simulink model "NumSim_standard_eVTOL"  (R2024b)
settings: Solver=ode14x  StartTime=0.0  StopTime=250  FixedStep=0.005  RelTol=1e-3
values from neighbouring files (symbols this model uses):
  aDl =     [initdata.mat]
  aDr =     [initdata.mat]
  aDyn =     [initdata.mat]
  Airport = init_airport('PHNL')    [initdata_HIL_eVTOL.m]
  aLat =     [initdata.mat]
  aLon =     [initdata.mat]
  D = Prop.D    [EOM_dt_MC.m]    (also in EOM_get_alf_dt_de_prop_evtol.m = CD * QS)
  dt0 = X(2)    [EOM_get_alf_dt_de_prop_evtol.m]    (also in initdata.mat = 0.258252593971; initdata_HIL_eVTOL.m = EOM_dt_MC)
  EAS0 = TAS0 / EAS2TAS    [initdata_HIL_eVTOL.m]
  FCS = init_FCS    [initdata_HIL_eVTOL.m]
  General = init_layoutdata    [EOM_dt_MC.m]    (also in build_optimized_CA.m; initdata.mat = ; initdata_HIL_eVTOL.m)
  h0 = Con(1)    [EOM_get_alf_dt_de_prop_evtol.m]    (also in initdata.mat = 450; initdata_HIL_eVTOL.m = 50)
  mass = Con(3)    [EOM_get_alf_dt_de_prop_evtol.m]    (also in initdata.mat = 2255.54; initdata_HIL_eVTOL.m = 7)
  Motor = init_motor_evtol    [EOM_dt_MC.m]    (also in initdata.mat = []; initdata_HIL_eVTOL.m)
  Prop = init_propeller_evtol_new    [EOM_dt_MC.m]    (also in initdata_HIL_eVTOL.m)
  R2D = 180/pi    (= 57.2957795131)    [EOM_get_alf_dt_de_prop_evtol.m]    (also in init_FCS.m; init_aerodata_evtol.m; init_airport.m; initdata.mat)
  theta0 = -0.0510981441662    [initdata.mat]
undefined symbols (not defined in the file or in its folder): A1, aDa, aDe, asbhl20env, B1, C1, de0, Earth, Environment, InitData, Kd, Kp, magnitude, Tc, WGS84
libraries: simulink_extras x26, simulink x18, slpidlib x14, vrlib x8, matrix_library x6, sharedutil x6, sharedtransform x5, aerolibwindfilters x4, aerolibatmos2 x3, aerolibobsolete x2, aerolibactuator x2, aerolibasang x2
(part 3 of 7)

== system NumSim_standard_eVTOL/Energy & Power/thrust_5/Motor ==
  P_shaft : Inport
  dt : Inport  Port=2
  V : Inport  Port=3
  rpm0 : Inport  Port=4
  rho : Inport  Port=5
  rpm_grid : Inport  Port=6
  Constant : Constant  Value=Motor.Ue
  Constant1 : Constant  Value=Motor.Re
  Constant2 : Constant  Value=Motor.Rm
  Constant3 : Constant  Value=Motor.KE
  Constant4 : Constant  Value=Motor.KT  VectorParams1D=off
  Constant5 : Constant  Value=Motor.Im0
  Constant6 : Constant  Value=0
  D^5 : Constant  Value=5
  Diameter : Constant  Value=Prop.D
  Diameter1 : Constant  Value=Prop.D
  Divide : Product  Inputs=*//
  Ea : Sum  Inputs=+-
  Gain1 : Gain  Gain=30/pi
  Gain2 : Gain  Gain=pi/30
  Gain3 : Gain  Gain=1/60
  Gain4 : Gain  Gain=1/(2*pi)
  Im : Sum
  Integrator : Integrator  InitialConditionSource=external  InitialCondition=600
  Ix : Constant  Value=Prop.Ix
  J : Product  Inputs=*//
  Manual Switch : ManualSwitch
  Math Function : Math  Operator=magnitude^2  SignedPower=on
  Math Function3 : Math  Operator=pow  SignedPower=on
  Math Function4 : Math  Operator=pow  SignedPower=on
  Memory : Memory  InitialCondition=0.1
  N(rpm) : Product  Inputs=*/
  N(rpm)1 : Product  Inputs=/*
  P Scope : Scope  NumInputPorts=2
  P_sp : Product  Inputs=4
  Product1 : Product
  Product2 : Product
  Q : Product  Inputs=4
  RPM 5 : Scope
  Saturation : Saturate  UpperLimit=1047.2  LowerLimit=0.1
  Scope : Scope
  Sum : Sum  Inputs=|+-
  Ueo : Product
  Um : Sum  Inputs=+-
  get CP : Lookup_n-D  BreakpointsForDimension1=Prop.J  BreakpointsForDimension2=Prop.rpm_grid  IndexSearchMethod=Linear search  BeginIndexSearchUsingPreviousIndexResult=on  Table=Prop.CP  RndMeth=Simplest
      settings: InputPortMap=u0,u1
  "n^3 " : Constant  Value=3
  rpm : Outport  VectorParamsAs1DForOutWhenUnconnected=off
  wires:
  Saturation/1 -> Gain1/1, Divide/2
  Gain2/1 -> Integrator/2
  rpm0/1 -> Manual Switch/1
  Gain1/1 -> rpm/1, RPM 5/1  "rpm"
  Sum/1 -> Divide/1  "DP"
  Divide/1 -> Integrator/1  "omega_dot"
  dt/1 -> Ueo/1
  Integrator/1 -> Saturation/1  "omega"
  P_sp/1 -> Scope/1, P Scope/1, Sum/1
  P_shaft/1 -> P Scope/2, Sum/2
  Ix/1 -> Divide/3
  Constant/1 -> Ueo/2
  Ueo/1 -> Um/1
  Product1/1 -> Um/2
  Constant1/1 -> Product1/1
  Um/1 -> Ea/1
  Product2/1 -> Ea/2
  Constant2/1 -> Product2/1
  Ea/1 -> N(rpm)/1
  Constant3/1 -> N(rpm)/2
  Diameter/1 -> J/2
  V/1 -> J/1
  N(rpm)/1 -> Gain3/1
  J/1 -> get CP/1
  rpm_grid/1 -> get CP/2
  Gain4/1 -> Q/2  "CQ"
  D^5/1 -> Math Function4/2
  Diameter1/1 -> Math Function4/1
  Math Function/1 -> Q/3  "n^2"
  Q/1 -> N(rpm)1/2
  Constant4/1 -> N(rpm)1/1
  N(rpm)1/1 -> Im/1
  Constant5/1 -> Im/2
  Im/1 -> Product1/2, Product2/2
  rho/1 -> Q/1, P_sp/3  "rho"
  Math Function3/1 -> P_sp/2  "n^3"
  "n^3 "/1 -> Math Function3/2
  Math Function4/1 -> Q/4, P_sp/4  "D^5"
  get CP/1 -> Gain4/1, P_sp/1  "CP"
  Constant6/1 -> Manual Switch/2
  Manual Switch/1 -> Gain2/1
  Gain3/1 -> Memory/1  "rps"
  Memory/1 -> J/3, Math Function3/1, Math Function/1

== system NumSim_standard_eVTOL/Energy & Power/thrust_5/Propeller  ==
  rpm : Inport
  V : Inport  Port=2
  rho : Inport  Port=3
  D^5 : Constant  Value=5
  Diameter : Constant  Value=Prop.D
  Divide : Product  Inputs=4
  Divide2 : Product  Inputs=4
  Divide3 : Product  Inputs=**/
  Gain : Gain  Gain=1/60
  Math Function : Math  Operator=magnitude^2  SignedPower=on
  Math Function1 : Math  Operator=magnitude^2  SignedPower=on
  Math Function2 : Math  Operator=magnitude^2  SignedPower=on
  Math Function3 : Math  Operator=pow  SignedPower=on
  Math Function4 : Math  Operator=pow  SignedPower=on
  Scope{,1..4} (5 alike) : Scope
  Subsystem : Subsystem
  get CP : Lookup_n-D  BreakpointsForDimension1=Prop.J  BreakpointsForDimension2=Prop.rpm_grid  IndexSearchMethod=Linear search  BeginIndexSearchUsingPreviousIndexResult=on  Table=Prop.CP  RndMeth=Simplest
      settings: InputPortMap=u0,u1
  get CT : Lookup_n-D  BreakpointsForDimension1=Prop.J  BreakpointsForDimension2=Prop.rpm_grid  IndexSearchMethod=Linear search  BeginIndexSearchUsingPreviousIndexResult=on  Table=Prop.CT  RndMeth=Simplest
      settings: InputPortMap=u0,u1
  "n^3 " : Constant  Value=3
  P_plr (w) : Outport  VectorParamsAs1DForOutWhenUnconnected=off
  T (N) : Outport  Port=2  VectorParamsAs1DForOutWhenUnconnected=off
  eta_p : Outport  Port=3  VectorParamsAs1DForOutWhenUnconnected=off
  wires:
  Divide2/1 -> P_plr (w)/1, Scope/1
  Divide3/1 -> eta_p/1  "eta_p"
  D^5/1 -> Math Function4/2
  Math Function4/1 -> Divide2/4
  "n^3 "/1 -> Math Function3/2
  Math Function3/1 -> Divide2/3
  get CP/1 -> Divide3/3, Divide2/1, Scope3/1
  Subsystem/1(J) -> Scope2/1, get CT/1, Divide3/1, get CP/1
  Divide/1 -> Scope1/1, T (N)/1
  Math Function2/1 -> Divide/4  "D^4"
  Math Function1/1 -> Math Function2/1
  Diameter/1 -> Math Function1/1, Math Function4/1
  Math Function/1 -> Divide/3  "n^2"
  Gain/1 -> Math Function3/1, Math Function/1
  rho/1 -> Divide/2, Divide2/2
  get CT/1 -> Divide3/2, Divide/1, Scope4/1
  V/1 -> Subsystem/1(V)
  rpm/1 -> get CP/2, get CT/2, Gain/1, Subsystem/2(rpm)

== system NumSim_standard_eVTOL/Energy & Power/thrust_6/Motor ==
  P_shaft : Inport
  dt : Inport  Port=2
  V : Inport  Port=3
  rpm0 : Inport  Port=4
  rho : Inport  Port=5
  rpm_grid : Inport  Port=6
  Constant : Constant  Value=Motor.Ue
  Constant1 : Constant  Value=Motor.Re
  Constant2 : Constant  Value=Motor.Rm
  Constant3 : Constant  Value=Motor.KE
  Constant4 : Constant  Value=Motor.KT  VectorParams1D=off
  Constant5 : Constant  Value=Motor.Im0
  Constant6 : Constant  Value=0
  D^5 : Constant  Value=5
  Diameter : Constant  Value=Prop.D
  Diameter1 : Constant  Value=Prop.D
  Divide : Product  Inputs=*//
  Ea : Sum  Inputs=+-
  Gain1 : Gain  Gain=30/pi
  Gain2 : Gain  Gain=pi/30
  Gain3 : Gain  Gain=1/60
  Gain4 : Gain  Gain=1/(2*pi)
  Im : Sum
  Integrator : Integrator  InitialConditionSource=external  InitialCondition=600
  Ix : Constant  Value=Prop.Ix
  J : Product  Inputs=*//
  Manual Switch : ManualSwitch
  Math Function : Math  Operator=magnitude^2  SignedPower=on
  Math Function3 : Math  Operator=pow  SignedPower=on
  Math Function4 : Math  Operator=pow  SignedPower=on
  Memory : Memory  InitialCondition=0.1
  N(rpm) : Product  Inputs=*/
  N(rpm)1 : Product  Inputs=/*
  P Scope : Scope  NumInputPorts=2
  P_sp : Product  Inputs=4
  Product1 : Product
  Product2 : Product
  Q : Product  Inputs=4
  RPM 6 : Scope
  Saturation : Saturate  UpperLimit=1047.2  LowerLimit=0.1
  Scope : Scope
  Sum : Sum  Inputs=|+-
  Ueo : Product
  Um : Sum  Inputs=+-
  get CP : Lookup_n-D  BreakpointsForDimension1=Prop.J  BreakpointsForDimension2=Prop.rpm_grid  IndexSearchMethod=Linear search  BeginIndexSearchUsingPreviousIndexResult=on  Table=Prop.CP  RndMeth=Simplest
      settings: InputPortMap=u0,u1
  "n^3 " : Constant  Value=3
  rpm : Outport  VectorParamsAs1DForOutWhenUnconnected=off
  wires:
  Saturation/1 -> Gain1/1, Divide/2
  Gain2/1 -> Integrator/2
  rpm0/1 -> Manual Switch/1
  Gain1/1 -> rpm/1, RPM 6/1  "rpm"
  Sum/1 -> Divide/1  "DP"
  Divide/1 -> Integrator/1  "omega_dot"
  dt/1 -> Ueo/1
  Integrator/1 -> Saturation/1  "omega"
  P_sp/1 -> Scope/1, P Scope/1, Sum/1
  P_shaft/1 -> P Scope/2, Sum/2
  Ix/1 -> Divide/3
  Constant/1 -> Ueo/2
  Ueo/1 -> Um/1
  Product1/1 -> Um/2
  Constant1/1 -> Product1/1
  Um/1 -> Ea/1
  Product2/1 -> Ea/2
  Constant2/1 -> Product2/1
  Ea/1 -> N(rpm)/1
  Constant3/1 -> N(rpm)/2
  Diameter/1 -> J/2
  V/1 -> J/1
  N(rpm)/1 -> Gain3/1
  J/1 -> get CP/1
  rpm_grid/1 -> get CP/2
  Gain4/1 -> Q/2  "CQ"
  D^5/1 -> Math Function4/2
  Diameter1/1 -> Math Function4/1
  Math Function/1 -> Q/3  "n^2"
  Q/1 -> N(rpm)1/2
  Constant4/1 -> N(rpm)1/1
  N(rpm)1/1 -> Im/1
  Constant5/1 -> Im/2
  Im/1 -> Product1/2, Product2/2
  rho/1 -> Q/1, P_sp/3  "rho"
  Math Function3/1 -> P_sp/2  "n^3"
  "n^3 "/1 -> Math Function3/2
  Math Function4/1 -> Q/4, P_sp/4  "D^5"
  get CP/1 -> Gain4/1, P_sp/1  "CP"
  Constant6/1 -> Manual Switch/2
  Manual Switch/1 -> Gain2/1
  Gain3/1 -> Memory/1  "rps"
  Memory/1 -> J/3, Math Function3/1, Math Function/1

== system NumSim_standard_eVTOL/Energy & Power/thrust_6/Propeller  ==
  rpm : Inport
  V : Inport  Port=2
  rho : Inport  Port=3
  D^5 : Constant  Value=5
  Diameter : Constant  Value=Prop.D
  Divide : Product  Inputs=4
  Divide2 : Product  Inputs=4
  Divide3 : Product  Inputs=**/
  Gain : Gain  Gain=1/60
  Math Function : Math  Operator=magnitude^2  SignedPower=on
  Math Function1 : Math  Operator=magnitude^2  SignedPower=on
  Math Function2 : Math  Operator=magnitude^2  SignedPower=on
  Math Function3 : Math  Operator=pow  SignedPower=on
  Math Function4 : Math  Operator=pow  SignedPower=on
  Scope{,1..4} (5 alike) : Scope
  Subsystem : Subsystem
  get CP : Lookup_n-D  BreakpointsForDimension1=Prop.J  BreakpointsForDimension2=Prop.rpm_grid  IndexSearchMethod=Linear search  BeginIndexSearchUsingPreviousIndexResult=on  Table=Prop.CP  RndMeth=Simplest
      settings: InputPortMap=u0,u1
  get CT : Lookup_n-D  BreakpointsForDimension1=Prop.J  BreakpointsForDimension2=Prop.rpm_grid  IndexSearchMethod=Linear search  BeginIndexSearchUsingPreviousIndexResult=on  Table=Prop.CT  RndMeth=Simplest
      settings: InputPortMap=u0,u1
  "n^3 " : Constant  Value=3
  P_plr (w) : Outport  VectorParamsAs1DForOutWhenUnconnected=off
  T (N) : Outport  Port=2  VectorParamsAs1DForOutWhenUnconnected=off
  eta_p : Outport  Port=3  VectorParamsAs1DForOutWhenUnconnected=off
  wires:
  Divide2/1 -> P_plr (w)/1, Scope/1
  Divide3/1 -> eta_p/1  "eta_p"
  D^5/1 -> Math Function4/2
  Math Function4/1 -> Divide2/4
  "n^3 "/1 -> Math Function3/2
  Math Function3/1 -> Divide2/3
  get CP/1 -> Divide3/3, Divide2/1, Scope3/1
  Subsystem/1(J) -> Scope2/1, get CT/1, Divide3/1, get CP/1
  Divide/1 -> Scope1/1, T (N)/1
  Math Function2/1 -> Divide/4  "D^4"
  Math Function1/1 -> Math Function2/1
  Diameter/1 -> Math Function1/1, Math Function4/1
  Math Function/1 -> Divide/3  "n^2"
  Gain/1 -> Math Function3/1, Math Function/1
  rho/1 -> Divide/2, Divide2/2
  get CT/1 -> Divide3/2, Divide/1, Scope4/1
  V/1 -> Subsystem/1(V)
  rpm/1 -> get CP/2, get CT/2, Gain/1, Subsystem/2(rpm)

== system NumSim_standard_eVTOL/Environment/Wind Models/Dryden Wind Turbulence Model (Continuous (+q -r)) ==
  Altitude : Inport  Unit=m
  Airspeed : Inport  Port=2  Unit=m/s
  DCM : Inport  Port=3  Unit=1  PortDimensions=[3 3]
  (u,v,w) : Selector  InputPortWidth=4  IndexOptions=Index vector (dialog)  Indices=[1 2 3]  OutputSizes=1
  Angle Conversion : Subsystem
  Bus Creator : BusCreator  Inputs=3
  Cast : DataTypeConversion  SaturateOnIntegerOverflow=off  RndMeth=Floor
  Cast To Double{,1..4} (5 alike) : DataTypeConversion  OutDataTypeStr=double  SaturateOnIntegerOverflow=off  RndMeth=Floor
  Disallow CGS : UnitConfiguration  UnitSystemsStr=English,SI,SI (extended)  AllowAllUnitSystems=off
  Filters on angular rates : Subsystem  mask(Angular Rates){}
  Filters on velocities : aerolibwindfilters/Dryden Continuous Filters  SystemSampleTime=-1  VariantActivationTime=update diagram  AllowFlexibleInterface=on  Latency=0  AutoFrameSizeCalculation=off
  Length Conversion : Subsystem
  Length Conversion1 : Subsystem
  Mux : Mux  Inputs=3
  Mux1 : Mux  Inputs=3
  RMS turbulence intensities : Subsystem
  Select angular rates : Subsystem
  Select velocities : Subsystem
  Turbulence scale lengths : Subsystem
  Unit Conversion : UnitConversion  OutputType=Inherit: Inherit via back propagation
  Velocity Conversion : Subsystem
  Velocity Conversion2 : Subsystem
  White Noise : aerolibcommonsys/Tunable White Noise  pwr=[1 1 1 1]*pi  Ts=ts  seed=Seed
  Wind direction : Constant  Value=Wdeg
  Windspeed at 20ft (6m) : Constant  Value=W20
  Wingspan : Constant  Value=Wingspan
  p : Selector  InputPortWidth=4  IndexOptions=Index vector (dialog)  Indices=[4]  OutputSizes=1
  ug,vg,wg : Outport  Unit=m/s  VectorParamsAs1DForOutWhenUnconnected=off
  pg,qg,rg : Outport  Port=2  VectorParamsAs1DForOutWhenUnconnected=off
  wires:
  Cast To Double4/1 -> Velocity Conversion/1(in)
  Airspeed/1 -> Cast To Double4/1
  Cast To Double3/1 -> Length Conversion1/1(in)
  Wingspan/1 -> Cast To Double3/1
  Cast To Double2/1 -> Length Conversion/1(in)
  Cast To Double1/1 -> Angle Conversion/1(in)
  Cast To Double/1 -> Bus Creator/1  "DCM"
  Mux1/1 -> Cast/1
  Cast/1 -> pg,qg,rg/1
  (u,v,w)/1 -> Filters on velocities/1
  Unit Conversion/1 -> ug,vg,wg/1
  Velocity Conversion/1(out) -> Filters on angular rates/3(V), Filters on velocities/8
  Angle Conversion/1(out) -> Bus Creator/2  "Wdeg"
  Length Conversion1/1(out) -> Filters on angular rates/7(wingspan)
  Bus Creator/1 -> Select angular rates/4("DCM, altitude, Wdeg"), Select velocities/1("DCM, altitude, Wdeg")
  DCM/1 -> Cast To Double/1  "DCM"
  Wind direction/1 -> Cast To Double1/1
  Select angular rates/3(rgw) -> Mux1/3
  Select angular rates/2(qgw) -> Mux1/2
  Select angular rates/1(pgw) -> Mux1/1
  Select velocities/3(wgw) -> Mux/3
  Select velocities/2(vgw) -> Mux/2
  Select velocities/1(ugw) -> Mux/1
  Velocity Conversion2/1(out) -> RMS turbulence intensities/2(Windspeed at 20ft (6m))
  Windspeed at 20ft (6m)/1 -> Velocity Conversion2/1(in)
  RMS turbulence intensities/2(sigma_vg) -> Filters on velocities/6
  Filters on velocities/3 -> Filters on angular rates/2(wg), Select velocities/4(wgw_h&l)  "wgw"
  Filters on velocities/2 -> Filters on angular rates/1(vg), Select velocities/3(vgw_h&l)  "vgw"
  RMS turbulence intensities/1("sigma_ug ") -> Filters on velocities/5
  Filters on velocities/1 -> Select velocities/2(ugw_h&l)  "ugw"
  Filters on angular rates/3(rgw) -> Select angular rates/3(rgw_h&l)  "rgw"
  Filters on angular rates/2(qgw) -> Select angular rates/2(qgw_h&l)  "qgw"
  Filters on angular rates/1(pgw) -> Select angular rates/1(pgw_h&l)  "pgw"
  RMS turbulence intensities/3(sigma_wg) -> Filters on angular rates/5(sigma_w), Filters on velocities/7
  Turbulence scale lengths/3(L_wg) -> Filters on angular rates/4(Lw), Filters on velocities/4
  Turbulence scale lengths/1(L_ug) -> Filters on velocities/2
  Altitude/1 -> Cast To Double2/1
  Mux/1 -> Unit Conversion/1
  White Noise/1 -> (u,v,w)/1, p/1
  p/1 -> Filters on angular rates/6(Noise)
  Length Conversion/1(out) -> Bus Creator/3, RMS turbulence intensities/1(Altitude), Turbulence scale lengths/1(Altitude)  "altitude"
  Turbulence scale lengths/2(L_vg) -> Filters on velocities/3

== system NumSim_standard_eVTOL/FCS/FW/Flare ==
  note: In my paper:
      | KHDot_Flare=0.024
      | KH_Flare=0.037
  H : Inport
  HDot : Inport  Port=2
  Enable : EnablePort
  Divide : Product  Inputs=*/
  Divide1 : Product  Inputs=**
  Gain : Gain
  HDot_Flare V=11 : Constant  Value=-0.57
  HDot_Flare V=12 : Constant  Value=-0.62
  HDot_TD : Constant  Value=-0.2
  H_Flare : Constant  Value=501.4
  H_TD : Constant  Value=500.4
  Integrator : Integrator
  KHDot_flare : Gain  Gain=0.6
  KH_flare : Gain  Gain=1.2
  Sum : Sum  Inputs=|++
  Sum1 : Sum  Inputs=|++
  Sum2 : Sum  Inputs=|+-
  Sum3 : Sum  Inputs=-+|
  Sum4 : Sum  Inputs=|+-
  Sum5 : Sum  Inputs=|+-
  Sum6 : Sum  Inputs=|++
  Transfer Fcn : TransferFcn  Numerator=[10 3]  Denominator=[1 3]
  dHdot Scope : Scope  NumInputPorts=2
  glide angle : Constant  Value=-3/57.3
  thetac : Outport  VectorParamsAs1DForOutWhenUnconnected=off
  wires:
  HDot/1 -> dHdot Scope/2, Sum3/1
  Sum3/1 -> KH_flare/1, KHDot_flare/1  "dHDot"
  Divide/1 -> Gain/1
  KH_flare/1 -> Integrator/1
  Sum/1 -> Sum6/1, Transfer Fcn/1
  Sum1/1 -> dHdot Scope/1, Sum3/2  "HDot_c"
  KHDot_flare/1 -> Sum/1
  Integrator/1 -> Sum/2
  Transfer Fcn/1 -> ?  "thetac"
  H_TD/1 -> Sum5/2, Sum4/2
  HDot_Flare V=11/1 -> Sum2/1
  H/1 -> Sum5/1
  Sum2/1 -> Divide/1
  HDot_TD/1 -> Sum2/2, Sum1/2
  Sum4/1 -> Divide/2
  H_Flare/1 -> Sum4/1
  Gain/1 -> Divide1/1
  Divide1/1 -> Sum1/1
  Sum5/1 -> Divide1/2
  Sum6/1 -> thetac/1
  glide angle/1 -> Sum6/2

== system NumSim_standard_eVTOL/FCS/FW/L1 guidance ==
  L1Mod : Inport
  L1 : Inport  Port=2
  R_circle : Inport  Port=3
  SensorData : Inport  Port=4
  NAVData : Inport  Port=5
  Bus Selector1 : BusSelector  OutputSignals=d,chi_WP
  Bus Selector3 : BusSelector  OutputSignals=Ve,chi
  Divide : Product  Inputs=*/
  Divide1 : Product  Inputs=*/
  Divide2 : Product  Inputs=***
  Divide3 : Product  Inputs=/*
  Divide4 : Product  Inputs=*/
  Dot Product : DotProduct  OutDataTypeStr=Inherit: Inherit via internal rule
  Gain : Gain  Gain=2
  Gain1 : Gain
  Gain2 : Gain  Gain=1/2
  Gain3 : Gain
  Multiport Switch : MultiPortSwitch  Inputs=2  SaturateOnIntegerOverflow=off  InputSameDT=off
  Radians to Degrees1 : simulink_extras/Transformations/Radians to Degrees
  Radians to Degrees2 : simulink_extras/Transformations/Radians to Degrees
  Radians to Degrees6 : simulink_extras/Transformations/Radians to Degrees
  Saturation : Saturate  UpperLimit=5/57.3  LowerLimit=-5/57.3
  Sqrt : Sqrt
  Sum : Sum  Inputs=|-+
  Sum1 : Sum  Inputs=|-+
  Sum2 : Sum  Inputs=|++
  Trigonometric Function : Trigonometry  Operator=asin
  Trigonometric Function1 : Trigonometry
  Trigonometric Function2 : Trigonometry  Operator=atan
  V : Scope
  "[+-0.7072]" : Saturate  UpperLimit=0.7072  LowerLimit=-0.7072
  ay : Scope
  chi_tr scp : Scope
  d scp : Scope
  eta1 scp : Scope
  eta{2..8} (7 alike) : Scope
  g : Constant  Value=9.8
  phic scp : Scope
  yc : Constant  Value=0
  phi_c : Outport  VectorParamsAs1DForOutWhenUnconnected=off
  eta1 : Outport  Port=2  VectorParamsAs1DForOutWhenUnconnected=off
  wires:
  [d] -> Sum/1
  Sum/1 -> d scp/1, Gain1/1  "d"
  L1/1 -> Gain2/1, eta5/1, Divide1/2, Divide/2
  Divide/1 -> "[+-0.7072]"/1
  Trigonometric Function/1 -> Sum2/1, Radians to Degrees2/1, eta1/1  "eta1"
  Trigonometric Function1/1 -> eta3/1, Multiport Switch/3  "sin(eta)_line"
  Divide1/1 -> eta4/1, Gain/1
  Gain/1 -> Divide2/3
  [V] -> Divide2/2, Divide2/1
  Divide2/1 -> Divide3/2, ay/1  "ay"
  g/1 -> Divide3/1
  Divide3/1 -> Trigonometric Function2/1
  Gain1/1 -> Divide/1
  Sum1/1 -> Gain3/1  "eta2"
  Sum2/1 -> Trigonometric Function1/1
  Multiport Switch/1 -> eta6/1, Divide1/1
  Gain2/1 -> Divide4/1
  Divide4/1 -> eta8/1, Multiport Switch/2  "sin(eta)_circle"
  R_circle/1 -> Divide4/2
  [chi] -> Sum1/1  "eta2"
  [chi_WP] -> Radians to Degrees1/1, Sum1/2
  L1Mod/1 -> Multiport Switch/1, eta7/1
  Radians to Degrees6/1 -> phic scp/1
  Radians to Degrees1/1 -> chi_tr scp/1
  Bus Selector1/1 -> [d]  "<d>"
  Bus Selector3/1 -> Dot Product/1, Dot Product/2  "<Ve>"
  NAVData/1 -> Bus Selector1/1
  Bus Selector3/2 -> [chi]  "<chi>"
  Bus Selector1/2 -> [chi_WP]  "<chi_WP>"
  SensorData/1 -> Bus Selector3/1
  yc/1 -> Sum/2
  Dot Product/1 -> Sqrt/1
  Sqrt/1 -> V/1, [V]
  Gain3/1 -> Sum2/2, eta2/1  "eta2"
  "[+-0.7072]"/1 -> Trigonometric Function/1
  Radians to Degrees2/1 -> eta1 scp/1
  Trigonometric Function2/1 -> Saturation/1
  Saturation/1 -> Radians to Degrees6/1, phi_c/1

== system NumSim_standard_eVTOL/FCS/FW/TECS ==
  FCSCMD : Inport
  SensorData : Inport  Port=2
  NAVCMD : Inport  Port=3
  Bus Selector1 : BusSelector  OutputSignals=Hc,TASc
  Bus Selector6 : BusSelector  OutputSignals=LonMod,Hc,Vc_TAS
  Bus Selector7 : BusSelector  OutputSignals=LLA_deg,Va
  Gain1 : Gain  Commented=on  Gain=-1
  Hc : Step  Commented=on  Time=20  Before=h0  After=h0+10  SampleTime=0
  Hc WP : Scope
  Manual Switch : ManualSwitch
  Manual Switch1 : ManualSwitch
  Selector3 : Selector  InputPortWidth=3  IndexOptions=Index vector (dialog)  Indices=3  OutputSizes=1
  Selector4 : Selector  Commented=on  InputPortWidth=3  IndexOptions=Index vector (dialog)  Indices=2  OutputSizes=1
  TECS PX4 & AP201 : Subsystem
  VC : Step  Commented=on  Time=0  Before=EAS0  After=EAS0  SampleTime=0
  Vc WP : Scope
  Vc_TAS scp : Scope
  thetac : Outport  VectorParamsAs1DForOutWhenUnconnected=off
  dt : Outport  Port=2  VectorParamsAs1DForOutWhenUnconnected=off
  wires:
  Selector3/1 -> TECS PX4 & AP201/2(h)
  Bus Selector6/1 -> TECS PX4 & AP201/1(LonMod)  "<LonMod>"
  SensorData/1 -> Bus Selector7/1
  Bus Selector7/2 -> TECS PX4 & AP201/3(V)  "<Va>"
  Selector4/1 -> Gain1/1
  Bus Selector7/1 -> Selector3/1  "<LLA_deg>"
  FCSCMD/1 -> Bus Selector6/1
  NAVCMD/1 -> Bus Selector1/1
  Manual Switch1/1 -> TECS PX4 & AP201/4(hc)
  Bus Selector6/3 -> Manual Switch/1  "<Vc_TAS>"
  Bus Selector1/2 -> Manual Switch/2, Vc WP/1  "<TASc>"
  Bus Selector1/1 -> Manual Switch1/2, Hc WP/1  "<Hc>"
  Bus Selector6/2 -> Manual Switch1/1  "<Hc>"
  TECS PX4 & AP201/2(thetac) -> thetac/1
  TECS PX4 & AP201/1(dt) -> dt/1
  Manual Switch/1 -> Vc_TAS scp/1, TECS PX4 & AP201/5(Vc)

== system NumSim_standard_eVTOL/FCS/FW/V hold//control ==
  note: VMod:
      | 1-cruise throt
      | 2-max throt
      | 3-min throt
      | 4-TECS
      | 5-Flare dt Fade
  CMDData : Inport
  SensorData : Inport  Port=2
  dt : Inport  Port=3
  Add : Sum
  Bus Selector1 : BusSelector  OutputSignals=Va
  Bus Selector4 : BusSelector  OutputSignals=VMod,Vc_TAS
  Compare To Constant : simulink/Logic and Bit Operations/Compare To Constant  relop===  const=1  OutDataTypeStr=uint8  ZeroCross=off
  Compare To Constant1 : simulink/Logic and Bit Operations/Compare To Constant  relop===  const=5  OutDataTypeStr=uint8  ZeroCross=off
  From1 : From  Commented=on  GotoTag=dtTrim  TagVisibility=scoped
      settings: CloseFcn=tagdialog Close
  From8 : From  Commented=on  GotoTag=dtTrim  TagVisibility=scoped
      settings: CloseFcn=tagdialog Close
  Multiport Switch : MultiPortSwitch  Inputs=5  SaturateOnIntegerOverflow=off  InputSameDT=off
  Saturation : Saturate  UpperLimit=1  LowerLimit=-1
  Saturation Dynamic : simulink/Discontinuities/Saturation Dynamic  Commented=on  OutMin=[]  OutMax=[]  OutDataTypeStr=Inherit: Same as second input  OutDataType=fixdt(1, 16)  OutScaling=2^-10  DoSatur=off
  Saturation1 : Saturate  UpperLimit=1.4  LowerLimit=-1.4
  Subsystem3 : Subsystem
  dt Fade at 0.1 / sec : Subsystem  TreatAsAtomicUnit=on
  dt=0 : Constant  Value=0
  dt=1 : Constant
  dtTrim : Constant  Value=0
  dvbar scp : Scope
  dvbar scp1 : Scope
  getV_bar : Subsystem
  dt cmd : Outport  VectorParamsAs1DForOutWhenUnconnected=off
  wires:
  Saturation/1 -> dt cmd/1  "dt"
  Bus Selector4/1 -> Compare To Constant1/1, Compare To Constant/1, Multiport Switch/1  "<VMod>"
  Compare To Constant/1 -> Subsystem3/1(VMod)
  dt=1/1 -> Multiport Switch/3
  From8/1 -> ?
  Subsystem3/1(dt_cmd) -> Saturation1/1, dvbar scp1/1
  Saturation1/1 -> dvbar scp/1, Multiport Switch/2
  Bus Selector4/2 -> getV_bar/2(V_c)  "<Vc_TAS>"
  getV_bar/1(V_bar) -> Subsystem3/2(dvbar)
  dt=0/1 -> Multiport Switch/6, Multiport Switch/4
  Compare To Constant1/1 -> dt Fade at 0.1 / sec/Enable
  Multiport Switch/1 -> dt Fade at 0.1 / sec/1(dt_ini), Saturation/1
  CMDData/1 -> Bus Selector4/1
  SensorData/1 -> Bus Selector1/1
  Bus Selector1/1 -> getV_bar/1(V)  "<Va>"
  dtTrim/1 -> Add/2
  dt/1 -> Add/1
  Add/1 -> Multiport Switch/5

== system NumSim_standard_eVTOL/FCS/FW/WayPoint Nav CMD ==
  note: FlightMod
      | 1-Ready
      | 2-TakeOff
      | 3-PullUp
      | 4-Climb
      | 5-Cruise, 5.1-circle, 5.2-line
      | 6-Return
      | 7-Approach
      | 8-Flare
      | 9-TouchDown
      | 10-Taxi
      | 11-GoAround
      | 12-Parachute
  SensorData : Inport
  Enable : EnablePort
  Bus Creator2 : BusCreator  Inputs=10
  Bus Selector3 : BusSelector  Commented=on  OutputSignals=IMUData.GPS_ENU,BaroData.V,BaroData.Ha
  Constant : Constant  Value=450
  Constant1 : Constant  Value=EAS0
  Constant2 : Constant  Commented=on  Value=1000
  Constant3 : Constant  Value=0
  Constant4 : Constant  Commented=on  Value=1000
  Constant5 : Constant  Value=0
  Constant6 : Constant  Commented=on  Value=0
  Constant7 : Constant  Value=450
  From : From  Commented=on  GotoTag=DS
  From3 : From  Commented=on  GotoTag=d_rem
  Gain : Gain  Gain=1/1.225
  Goto : Goto  Commented=on  GotoTag=DS
  Goto3 : Goto  Commented=on  GotoTag=d_rem
  Goto7 : Goto  Commented=on  GotoTag=dh_2traj
  ISA Atmosphere Model : aerolibatmos2/ISA Atmosphere Model  useExtended=off  action=Warning  custom=off  viscosityOut=off  g=9.80665  gamma=1.4  R=287.0531  L=0.0065  h_trop=11000  h_strat=20000  rho0=1.225  P0=101325  T0=288.15  h0=0  S=110.4  Tref=273.15  muref=1.716e-5
  Mission_ID : Constant  Value=0
  Mux1 : Mux  Inputs=6
  Product : Product  Inputs=*/
  Selector1 : Selector  Commented=on  InputPortWidth=3  IndexOptions=Index vector (dialog)  Indices=2  OutputSizes=1
  Selector2 : Selector  Commented=on  InputPortWidth=3  IndexOptions=Index vector (dialog)  Indices=1  OutputSizes=1
  Selector3 : Selector  Commented=on  InputPortWidth=3  IndexOptions=Index vector (dialog)  Indices=3  OutputSizes=1
  Sqrt : Sqrt
  Terminator : Terminator
  Terminator1 : Terminator
  Terminator2 : Terminator
  WP# : Constant
  NAVCMD : Outport  VectorParamsAs1DForOutWhenUnconnected=off
  wires:
  WP#/1 -> Mux1/5
  From/1 -> Bus Creator2/6  "DS"
  [d] -> Bus Creator2/4  "d"
  From3/1 -> Bus Creator2/5  "d_rem"
  Selector2/1 -> Mux1/2  "lon"
  Selector1/1 -> Mux1/1  "lat"
  Mux1/1 -> Bus Creator2/1  "UAVPos"
  [chi_WP] -> Bus Creator2/7  "chi_WP"
  Bus Creator2/1 -> NAVCMD/1
  [Hc] -> Bus Creator2/8  "Hc"
  [EASc] -> Bus Creator2/9  "EASc"
  SensorData/1 -> Bus Selector3/1
  Bus Selector3/2 -> Mux1/4  "<V>"
  Bus Selector3/1 -> Selector2/1, Selector3/1, Selector1/1  "<GPS_ENU>"
  Selector3/1 -> Mux1/3  "h"
  Constant2/1 -> Goto/1
  Constant3/1 -> [chi_WP]
  Constant5/1 -> [d]
  Constant4/1 -> Goto3/1
  Constant7/1 -> [H_WPB]
  Constant1/1 -> [EASc]
  Constant6/1 -> Goto7/1
  Constant/1 -> [Hc]
  Mission_ID/1 -> Mux1/6
  Bus Selector3/3 -> ISA Atmosphere Model/1  "<Ha>"
  ISA Atmosphere Model/1 -> Terminator/1
  ISA Atmosphere Model/2 -> Terminator1/1
  ISA Atmosphere Model/3 -> Terminator2/1
  ISA Atmosphere Model/4 -> [rho]
  [rho] -> Gain/1
  Gain/1 -> Sqrt/1
  [EASc] -> Product/1  "TASc"
  Sqrt/1 -> Product/2
  Product/1 -> [TASc]
  [TASc] -> Bus Creator2/10  "TASc"

== system NumSim_standard_eVTOL/FCS/FW/alpha limit ==
  alpha : Inport
  Add2 : Sum  Inputs=-+
  Compare To Constant : simulink/Logic and Bit Operations/Compare To Constant  relop=>=  const=0  OutDataTypeStr=uint8  ZeroCross=off
  Lookup Table : Lookup  InputValues=[7, 7.5, 8.0] ./57.3  Table=[-50, -120,-250]  SaturateOnIntegerOverflow=off
  Product : Product  RndMeth=Zero
  Saturation1 : Saturate  UpperLimit=inf  LowerLimit=0
  Scope1 : Scope
  Scope2 : Scope
  Subsystem : Subsystem
  limit alpha : Constant  Value=7/57.3
  de : Outport  VectorParamsAs1DForOutWhenUnconnected=off
  wires:
  Subsystem/1(Out1) -> Scope1/1, de/1
  limit alpha/1 -> Add2/1
  alpha/1 -> Add2/2, Lookup Table/1
  Add2/1 -> Compare To Constant/1, Saturation1/1, Scope2/1
  Saturation1/1 -> Product/1
  Compare To Constant/1 -> Subsystem/Enable
  Product/1 -> Subsystem/1(In1)
  Lookup Table/1 -> Product/2

== system NumSim_standard_eVTOL/FCS/FW/phi hold&control ==
  phic : Inport
  SensorData : Inport  Port=2
  Bus Selector1 : BusSelector  OutputSignals=Euler,pqr,Ab,Va
  Divide : Product  Inputs=*/
  Gain : Gain
  Gain1 : Gain  Gain=-1
  Integrator : Integrator  Commented=on  LimitOutput=on  UpperSaturationLimit=0.2  LowerSaturationLimit=-0.2
  Kp_dd : Gain  Commented=on  Gain=0.05
  Kphi : Gain  Gain=0.25
  Kpi_dd : Gain  Commented=on  Gain=0.005
  Kr1 : Gain  Gain=9.8
  Kr2 : Gain  Gain=0.3
  PID Controller : slpidlib/PID Controller  Controller=PI  Form=Parallel  TimeDomain=Continuous-time  UseExternalTs=off  SampleTime=-1  IntegratorMethod=Forward Euler  FilterMethod=Forward Euler  ControllerParametersSource=internal  P=0.025  I=0005  UseKiTs=off  D=0  UseExternalDerivativeSource=off  N=100  UseFilter=on  TunerSelectOption=Transfer Function Based (PID Tuner App)  InitialConditionSource=internal  InitialConditionForIntegrator=0  InitialConditionForFilter=0  DifferentiatorICPrevScaledInput=0  ExternalReset=none  TrackingMode=off  Kt=1  LimitOutput=on  SatLimitsSource=internal  UpperSaturationLimit=25/57.3  LowerSaturationLimit=-25/57.3  LinearizeAsGain=on  AntiWindupMode=none  Kb=1  LimitIntegrator=off  UpperIntegratorSaturationLimit=inf  LowerIntegratorSaturationLimit=-inf  POutMin=[]  POutMax=[]  IOutMin=[]  IOutMax=[]  DOutMin=[]  DOutMax=[]  NOutMin=[]  NOutMax=[]  SumOutMin=[]  SumOutMax=[]  SaturationOutMin=[]  SaturationOutMax=[]  PParamMin=[]  PParamMax=[]  IParamMin=[]  IParamMax=[]  DParamMin=[]  DParamMax=[]  NParamMin=[]  NParamMax=[]  KbParamMin=[]  KbParamMax=[]  KtParamMin=[]  KtParamMax=[]  KbOutMin=[]  KbOutMax=[]  KtOutMin=[]  KtOutMax=[]  IntegratorOutMin=[]  IntegratorOutMax=[]  FilterOutMin=[]  FilterOutMax=[]  SumI1OutMin=[]  SumI1OutMax=[]  SumI2OutMin=[]  SumI2OutMax=[]  SumI3OutMin=[]  SumI3OutMax=[]  SumI4OutMin=[]  SumI4OutMax=[]  SumDOutMin=[]  SumDOutMax=[]  DifferentiatorOutMin=[]  DifferentiatorOutMax=[]  FilterDiffOutCoefMin=[]  FilterDiffOutCoefMax=[]  ReciprocalOutMin=[]  ReciprocalOutMax=[]  SumDenOutMin=[]  SumDenOutMax=[]  SumNumOutMin=[]  SumNumOutMax=[]  DivideOutMin=[]  DivideOutMax=[]  UdiffTsProdOutMin=[]  UdiffTsProdOutMax=[]  NTsProdOutMin=[]  NTsProdOutMax=[]  UintegralTsProdOutMin=[]  UintegralTsProdOutMax=[]  UngainTsProdOutMin=[]  UngainTsProdOutMax=[]  ClampingZeroOutDataTypeStr=Inherit: Inherit via back propagation  ClampingZeroOutMin=[]  ClampingZeroOutMax=[]  FilterDenConstantOutDataTypeStr=Inherit: Inherit via back propagation  FilterDenConstantOutMin=[]  FilterDenConstantOutMax=[]  PCopyOutDataTypeStr=Inherit: Inherit via back propagation  PCopyOutMin=[]  PCopyOutMax=[]  NCopyOutDataTypeStr=Inherit: Inherit via back propagation  NCopyOutMin=[]  NCopyOutMax=[]  IntegratorContinuousStateAttributes=''  IntegratorStateMustResolveToSignalObject=off  IntegratorRTWStateStorageClass=Auto  FilterContinuousStateAttributes=''  FilterStateMustResolveToSignalObject=off  FilterRTWStateStorageClass=Auto  ParallelPVariant=InternalParameters  IdealPVariant=Disabled  IVariant=InternalParameters  DVariant=Disabled  IntegratorVariant=Continuous  SatVariant=Enabled  AWVariant=Passthrough  PCopyVariant=Disabled  TRVariant=Disabled  FdbkBlocksVariant=Forward  IdealPFdbkVariant=Disabled  SatFdbkVariant=Disabled  DerivativeFilterVariant=Disabled  NVariant=Disabled  NCopyVariant=Disabled_SignalSpec  FilterICVariant=Disabled  IntegratorICVariant=InternalICs  ExternalResetVariant=Disabled  TRSumVariant=Passthrough  SumFdbkVariant=Disabled  SumVariant=Sum_PI  TsampFilterVariant=InternalTs  TsampNgainVariant=Passthrough  TsampIntegralVariant=Disabled_SignalSpec  ExternalSaturationOutDataTypeStr=Inherit: Same as second input  DerivativeSourceVariant=Disabled  PreIntVariant=InternalPreInt
  Radians to Degrees1 : simulink_extras/Transformations/Radians to Degrees
  Saturation : Saturate  UpperLimit=inf  LowerLimit=1
  Scope : Scope
  Selector1 : Selector  InputPortWidth=3  IndexOptions=Index vector (dialog)  Indices=1  OutputSizes=1
  Selector2 : Selector  InputPortWidth=3  IndexOptions=Index vector (dialog)  Indices=1  OutputSizes=1
  Selector3 : Selector  InputPortWidth=3  IndexOptions=Index vector (dialog)  Indices=3  OutputSizes=1
  Selector4 : Selector  InputPortWidth=3  IndexOptions=Index vector (dialog)  Indices=2  OutputSizes=1
  Sum1 : Sum  Inputs=|+-
  Sum2 : Sum  Commented=on  Inputs=|++
  Sum4 : Sum  Inputs=|+-
  Sum5 : Sum  Inputs=|+-
  Tan : Trigonometry  Operator=tan
  da scp : Scope
  da : Outport  VectorParamsAs1DForOutWhenUnconnected=off
  dr : Outport  Port=2  VectorParamsAs1DForOutWhenUnconnected=off
  wires:
  phic/1 -> [phic]
  SensorData/1 -> Bus Selector1/1
  Bus Selector1/1 -> Selector1/1  "<Euler>"
  Selector1/1 -> [phi]
  Bus Selector1/2 -> Selector3/1, Selector2/1  "<pqr>"
  Selector2/1 -> [p]
  Selector3/1 -> [r]
  Bus Selector1/3 -> Selector4/1  "<Ab>"
  Selector4/1 -> [ay]
  [phic] -> Sum5/1
  [r] -> Kr2/1
  [p] -> Sum4/1
  Kr2/1 -> Sum1/1
  Integrator/1 -> Sum2/2
  Radians to Degrees1/1 -> da scp/1
  Kphi/1 -> Sum4/2  "pc"
  [phi] -> Sum5/2
  Kpi_dd/1 -> Integrator/1
  Sum4/1 -> Scope/1, PID Controller/1
  Sum5/1 -> Kphi/1
  Kp_dd/1 -> Sum2/1
  [phi] -> Tan/1
  Tan/1 -> Kr1/1
  Bus Selector1/4 -> [Va]  "<Va>"
  Kr1/1 -> Divide/1
  Saturation/1 -> Divide/2
  [Va] -> Saturation/1
  Divide/1 -> Sum1/2
  Gain/1 -> Radians to Degrees1/1, da/1
  Sum1/1 -> Gain1/1
  Gain1/1 -> dr/1
  PID Controller/1 -> Gain/1

== system NumSim_standard_eVTOL/FCS/FW/theta hold&control ==
  note: LonMod:
      | 1-theta hold
      | 2-height hold
      | 3-gamma control
      | 4-landing flare control
      | 5-TakeOff
  CMDData : Inport
  SensorData : Inport  Port=2
  thetac : Inport  Port=3
  Add1 : Sum  Inputs=|-+
  Add2 : Sum  Inputs=|+-
  Add4 : Sum  Commented=on
  Bus Selector1 : BusSelector  OutputSignals=LonMod
  Bus Selector2 : BusSelector  OutputSignals=Euler,pqr
  Constant : Constant  Value=0
  Data Type Conversion : DataTypeConversion  OutDataTypeStr=boolean  SaturateOnIntegerOverflow=off  RndMeth=Floor
  Integrator : Integrator  Commented=on  ExternalReset=either  LimitOutput=on  UpperSaturationLimit=5  LowerSaturationLimit=-5
  Memory : Memory
  OMEGA : Gain  Gain=1.8
  PID Controller : slpidlib/PID Controller  Controller=PI  Form=Parallel  TimeDomain=Continuous-time  UseExternalTs=off  SampleTime=-1  IntegratorMethod=Forward Euler  FilterMethod=Forward Euler  ControllerParametersSource=internal  P=0.5  I=0.02  UseKiTs=off  D=0  UseExternalDerivativeSource=off  N=100  UseFilter=on  TunerSelectOption=Transfer Function Based (PID Tuner App)  InitialConditionSource=internal  InitialConditionForIntegrator=-0.022  InitialConditionForFilter=0  DifferentiatorICPrevScaledInput=0  ExternalReset=either  TrackingMode=off  Kt=1  LimitOutput=on  SatLimitsSource=internal  UpperSaturationLimit=25/57.3  LowerSaturationLimit=-25/57.3  LinearizeAsGain=on  AntiWindupMode=clamping  Kb=1  LimitIntegrator=off  UpperIntegratorSaturationLimit=inf  LowerIntegratorSaturationLimit=-inf  POutMin=[]  POutMax=[]  IOutMin=[]  IOutMax=[]  DOutMin=[]  DOutMax=[]  NOutMin=[]  NOutMax=[]  SumOutMin=[]  SumOutMax=[]  SaturationOutMin=[]  SaturationOutMax=[]  PParamMin=[]  PParamMax=[]  IParamMin=[]  IParamMax=[]  DParamMin=[]  DParamMax=[]  NParamMin=[]  NParamMax=[]  KbParamMin=[]  KbParamMax=[]  KtParamMin=[]  KtParamMax=[]  KbOutMin=[]  KbOutMax=[]  KtOutMin=[]  KtOutMax=[]  IntegratorOutMin=[]  IntegratorOutMax=[]  FilterOutMin=[]  FilterOutMax=[]  SumI1OutMin=[]  SumI1OutMax=[]  SumI2OutMin=[]  SumI2OutMax=[]  SumI3OutMin=[]  SumI3OutMax=[]  SumI4OutMin=[]  SumI4OutMax=[]  SumDOutMin=[]  SumDOutMax=[]  DifferentiatorOutMin=[]  DifferentiatorOutMax=[]  FilterDiffOutCoefMin=[]  FilterDiffOutCoefMax=[]  ReciprocalOutMin=[]  ReciprocalOutMax=[]  SumDenOutMin=[]  SumDenOutMax=[]  SumNumOutMin=[]  SumNumOutMax=[]  DivideOutMin=[]  DivideOutMax=[]  UdiffTsProdOutMin=[]  UdiffTsProdOutMax=[]  NTsProdOutMin=[]  NTsProdOutMax=[]  UintegralTsProdOutMin=[]  UintegralTsProdOutMax=[]  UngainTsProdOutMin=[]  UngainTsProdOutMax=[]  ClampingZeroOutDataTypeStr=Inherit: Inherit via back propagation  ClampingZeroOutMin=[]  ClampingZeroOutMax=[]  FilterDenConstantOutDataTypeStr=Inherit: Inherit via back propagation  FilterDenConstantOutMin=[]  FilterDenConstantOutMax=[]  PCopyOutDataTypeStr=Inherit: Inherit via back propagation  PCopyOutMin=[]  PCopyOutMax=[]  NCopyOutDataTypeStr=Inherit: Inherit via back propagation  NCopyOutMin=[]  NCopyOutMax=[]  IntegratorContinuousStateAttributes=''  IntegratorStateMustResolveToSignalObject=off  IntegratorRTWStateStorageClass=Auto  FilterContinuousStateAttributes=''  FilterStateMustResolveToSignalObject=off  FilterRTWStateStorageClass=Auto  ParallelPVariant=InternalParameters  IdealPVariant=Disabled  IVariant=InternalParameters  DVariant=Disabled  IntegratorVariant=Continuous  SatVariant=Enabled  AWVariant=ContClampingParallel  PCopyVariant=Disabled  TRVariant=Disabled  FdbkBlocksVariant=Forward  IdealPFdbkVariant=Disabled  SatFdbkVariant=Disabled  DerivativeFilterVariant=Disabled  NVariant=Disabled  NCopyVariant=Disabled_SignalSpec  FilterICVariant=Disabled  IntegratorICVariant=InternalICs  ExternalResetVariant=ExternalReset  TRSumVariant=Passthrough  SumFdbkVariant=Disabled  SumVariant=Sum_PI  TsampFilterVariant=InternalTs  TsampNgainVariant=Passthrough  TsampIntegralVariant=Disabled_SignalSpec  ExternalSaturationOutDataTypeStr=Inherit: Same as second input  DerivativeSourceVariant=Disabled  PreIntVariant=InternalPreInt
  Radians to Degrees : simulink_extras/Transformations/Radians to Degrees
  Radians to Degrees1 : simulink_extras/Transformations/Radians to Degrees
  Saturation : Saturate  UpperLimit=25/57.3  LowerLimit=-25/57.3
  Scope : Scope
  Scope1 : Scope
  Scope5 : Scope
  Selector1 : Selector  InputPortWidth=3  IndexOptions=Index vector (dialog)  Indices=2  OutputSizes=1
  Selector2 : Selector  InputPortWidth=3  IndexOptions=Index vector (dialog)  Indices=2  OutputSizes=1
  Slon : MultiPortSwitch  Inputs=5  SaturateOnIntegerOverflow=off  InputSameDT=off
  Slon1 : MultiPortSwitch  Inputs=5  SaturateOnIntegerOverflow=off  InputSameDT=off
  "[-15,15]" : Saturate  UpperLimit=15/57.3  LowerLimit=-15/57.3
  "[-15,15]-" : Saturate  UpperLimit=15/57.3  LowerLimit=-15/57.3
  de0 in take-off : Constant  Value=-1/57.3
  kq : Gain  Commented=on  Gain=0.5
  kq1 : Gain
  kqi : Gain  Commented=on  Gain=0.02
  kqi2 : Gain  Gain=2
  qc limit : Saturate  UpperLimit=10/57.3  LowerLimit=-10/57.3
  thetac scp : Scope
  de : Outport  VectorParamsAs1DForOutWhenUnconnected=off
  wires:
  Bus Selector1/1 -> [LonMod]  "<LonMod>"
  CMDData/1 -> Bus Selector1/1
  Bus Selector2/2 -> Selector2/1  "<pqr>"
  Selector2/1 -> [q]
  SensorData/1 -> Bus Selector2/1
  thetac/1 -> [thetac]
  Selector1/1 -> [theta]
  Bus Selector2/1 -> Selector1/1  "<Euler>"
  Constant/1 -> Slon1/6
  "[-15,15]-"/1 -> Slon1/5
  [LonMod] -> Slon1/1, Slon/1
  Add2/1 -> OMEGA/1
  [theta] -> Add2/2
  [q] -> Add1/2
  OMEGA/1 -> Scope1/1, qc limit/1
  kq1/1 -> kqi2/1, Slon/4, Slon/3, Slon/2
  de0 in take-off/1 -> Slon/6
  kqi2/1 -> Slon/5
  Memory/1 -> Data Type Conversion/1
  qc limit/1 -> Add1/1  "qc"
  [thetac] -> "[-15,15]-"/1, "[-15,15]"/1
  Radians to Degrees/1 -> thetac scp/1
  "[-15,15]"/1 -> Slon1/4, Slon1/3, Slon1/2
  Integrator/1 -> kqi/1
  Slon1/1 -> Radians to Degrees/1, Memory/1, Add2/1
  Radians to Degrees1/1 -> Scope/1
  Slon/1 -> Saturation/1
  Saturation/1 -> Radians to Degrees1/1, de/1
  kq/1 -> Add4/1
  kqi/1 -> Add4/2
  Add1/1 -> PID Controller/1
  PID Controller/1 -> Scope5/1, kq1/1
  Data Type Conversion/1 -> PID Controller/2

== system NumSim_standard_eVTOL/FCS/FW/trim data ==
  H : Inport
  Gain : Gain  Gain=-0.00000005
  Sum : Sum  Inputs=|+-
  Sum1 : Sum  Inputs=|++
  phic1 : Constant  Value=theta0
  phic2 : Constant  Value=dt0
  phic3 : Constant  Value=h0
  phic9 : Constant  Value=de0
  deTrim : Outport  VectorParamsAs1DForOutWhenUnconnected=off
  dtTrim : Outport  Port=2  VectorParamsAs1DForOutWhenUnconnected=off
  thetaTrim : Outport  Port=3  VectorParamsAs1DForOutWhenUnconnected=off
  wires:
  phic1/1 -> thetaTrim/1
  phic2/1 -> dtTrim/1
  H/1 -> Sum/1
  phic3/1 -> Sum/2
  phic9/1 -> Sum1/2
  Sum1/1 -> deTrim/1
  Sum/1 -> Gain/1
  Gain/1 -> ?

== system NumSim_standard_eVTOL/FCS/MC/ADRC theta ==
  thetac : Inport
  theta : Inport  Port=2
  1/B : Gain  Gain=1/(-125)
  Constant : Constant  Value=[pi/4, 0, 0]
  Demux : Demux  Outputs=3
  ESO : Subsystem
  Gain : Gain  Gain=Kp
  Gain1 : Gain  Gain=Kd
  Mux : Mux  Inputs=2
  Radians to Degrees : simulink_extras/Transformations/Radians to Degrees
  Scope{,1..6} (7 alike) : Scope
  Sum : Sum  Inputs=|+-
  Sum1 : Sum  Inputs=|+-
  Sum2 : Sum  Inputs=|++
  Sum4 : Sum  Inputs=|+-
  TD : Subsystem
  consituous TD : Subsystem
  de : Outport
  wires:
  Demux/2 -> Sum1/2  "theta_dot"
  Sum1/1 -> Gain1/1
  1/B/1 -> Mux/1, de/1, Scope3/1
  theta/1 -> Mux/2
  ESO/1(x) -> ?
  Sum4/1 -> 1/B/1
  Sum2/1 -> Sum4/1  "u0"
  Demux/3 -> Sum4/2  "theta_dotdot"
  ESO/2(y) -> Demux/1
  Gain1/1 -> Scope2/1, Sum2/2
  Demux/1 -> Sum/2  "theta"
  Mux/1 -> ESO/1(u)
  thetac/1 -> consituous TD/1(v), TD/1(v)
  Gain/1 -> Scope1/1, Sum2/1
  Sum/1 -> Gain/1
  Radians to Degrees/1 -> Scope4/1
  Constant/1 -> ESO/2(x0)
  consituous TD/2(v2) -> Sum1/1, Scope/1
  consituous TD/1(v1) -> Sum/1, Radians to Degrees/1
  TD/2(v2) -> Scope5/1
  TD/1(v1) -> Scope6/1

== system NumSim_standard_eVTOL/FCS/MC/Height control ==
  Ve : Inport
  Xe : Inport  Port=2
  h_c : Inport  Port=3
  Demux5 : Demux  Outputs=3
  Demux6 : Demux  Outputs=3
  Gain : Gain  Gain=-1
  Gain4 : Gain  Gain=-1
  Gain5 : Gain  Gain=-1
  PID Controller : slpidlib/PID Controller  Controller=PID  Form=Parallel  TimeDomain=Continuous-time  UseExternalTs=off  SampleTime=-1  IntegratorMethod=Forward Euler  FilterMethod=Forward Euler  ControllerParametersSource=internal  P=0.3  I=0  UseKiTs=off  D=0  UseExternalDerivativeSource=off  N=100  UseFilter=on  TunerSelectOption=Transfer Function Based (PID Tuner App)  InitialConditionSource=internal  InitialConditionForIntegrator=0  InitialConditionForFilter=0  DifferentiatorICPrevScaledInput=0  ExternalReset=none  TrackingMode=off  Kt=1  LimitOutput=off  SatLimitsSource=internal  UpperSaturationLimit=inf  LowerSaturationLimit=-inf  LinearizeAsGain=on  AntiWindupMode=none  Kb=1  LimitIntegrator=off  UpperIntegratorSaturationLimit=inf  LowerIntegratorSaturationLimit=-inf  POutMin=[]  POutMax=[]  IOutMin=[]  IOutMax=[]  DOutMin=[]  DOutMax=[]  NOutMin=[]  NOutMax=[]  SumOutMin=[]  SumOutMax=[]  SaturationOutMin=[]  SaturationOutMax=[]  PParamMin=[]  PParamMax=[]  IParamMin=[]  IParamMax=[]  DParamMin=[]  DParamMax=[]  NParamMin=[]  NParamMax=[]  KbParamMin=[]  KbParamMax=[]  KtParamMin=[]  KtParamMax=[]  KbOutMin=[]  KbOutMax=[]  KtOutMin=[]  KtOutMax=[]  IntegratorOutMin=[]  IntegratorOutMax=[]  FilterOutMin=[]  FilterOutMax=[]  SumI1OutMin=[]  SumI1OutMax=[]  SumI2OutMin=[]  SumI2OutMax=[]  SumI3OutMin=[]  SumI3OutMax=[]  SumI4OutMin=[]  SumI4OutMax=[]  SumDOutMin=[]  SumDOutMax=[]  DifferentiatorOutMin=[]  DifferentiatorOutMax=[]  FilterDiffOutCoefMin=[]  FilterDiffOutCoefMax=[]  ReciprocalOutMin=[]  ReciprocalOutMax=[]  SumDenOutMin=[]  SumDenOutMax=[]  SumNumOutMin=[]  SumNumOutMax=[]  DivideOutMin=[]  DivideOutMax=[]  UdiffTsProdOutMin=[]  UdiffTsProdOutMax=[]  NTsProdOutMin=[]  NTsProdOutMax=[]  UintegralTsProdOutMin=[]  UintegralTsProdOutMax=[]  UngainTsProdOutMin=[]  UngainTsProdOutMax=[]  ClampingZeroOutDataTypeStr=Inherit: Inherit via back propagation  ClampingZeroOutMin=[]  ClampingZeroOutMax=[]  FilterDenConstantOutDataTypeStr=Inherit: Inherit via back propagation  FilterDenConstantOutMin=[]  FilterDenConstantOutMax=[]  PCopyOutDataTypeStr=Inherit: Inherit via back propagation  PCopyOutMin=[]  PCopyOutMax=[]  NCopyOutDataTypeStr=Inherit: Inherit via back propagation  NCopyOutMin=[]  NCopyOutMax=[]  IntegratorContinuousStateAttributes=''  IntegratorStateMustResolveToSignalObject=off  IntegratorRTWStateStorageClass=Auto  FilterContinuousStateAttributes=''  FilterStateMustResolveToSignalObject=off  FilterRTWStateStorageClass=Auto  ParallelPVariant=InternalParameters  IdealPVariant=Disabled  IVariant=InternalParameters  DVariant=InternalParameters  IntegratorVariant=Continuous  SatVariant=Disabled  AWVariant=Passthrough  PCopyVariant=Disabled  TRVariant=Disabled  FdbkBlocksVariant=Forward  IdealPFdbkVariant=Disabled  SatFdbkVariant=Disabled  DerivativeFilterVariant=ContFilter  NVariant=InternalParameters  NCopyVariant=Disabled  FilterICVariant=InternalICsFilter  IntegratorICVariant=InternalICs  ExternalResetVariant=Disabled  TRSumVariant=Passthrough  SumFdbkVariant=Disabled  SumVariant=Sum_PID  TsampFilterVariant=InternalTs  TsampNgainVariant=Passthrough  TsampIntegralVariant=Disabled_SignalSpec  ExternalSaturationOutDataTypeStr=Inherit: Same as second input  DerivativeSourceVariant=ErrorSignal  PreIntVariant=InternalPreInt
  PID Controller2 : slpidlib/PID Controller  Controller=PID  Form=Parallel  TimeDomain=Continuous-time  UseExternalTs=off  SampleTime=-1  IntegratorMethod=Forward Euler  FilterMethod=Forward Euler  ControllerParametersSource=internal  P=3  I=3  UseKiTs=off  D=1  UseExternalDerivativeSource=off  N=65.6590999771333  UseFilter=on  TunerSelectOption=Transfer Function Based (PID Tuner App)  InitialConditionSource=internal  InitialConditionForIntegrator=0  InitialConditionForFilter=0  DifferentiatorICPrevScaledInput=0  ExternalReset=none  TrackingMode=off  Kt=1  LimitOutput=on  SatLimitsSource=internal  UpperSaturationLimit=1.8  LowerSaturationLimit=-1.8  LinearizeAsGain=on  AntiWindupMode=clamping  Kb=1  LimitIntegrator=off  UpperIntegratorSaturationLimit=inf  LowerIntegratorSaturationLimit=-inf  POutMin=[]  POutMax=[]  IOutMin=[]  IOutMax=[]  DOutMin=[]  DOutMax=[]  NOutMin=[]  NOutMax=[]  SumOutMin=[]  SumOutMax=[]  SaturationOutMin=[]  SaturationOutMax=[]  PParamMin=[]  PParamMax=[]  IParamMin=[]  IParamMax=[]  DParamMin=[]  DParamMax=[]  NParamMin=[]  NParamMax=[]  KbParamMin=[]  KbParamMax=[]  KtParamMin=[]  KtParamMax=[]  KbOutMin=[]  KbOutMax=[]  KtOutMin=[]  KtOutMax=[]  IntegratorOutMin=[]  IntegratorOutMax=[]  FilterOutMin=[]  FilterOutMax=[]  SumI1OutMin=[]  SumI1OutMax=[]  SumI2OutMin=[]  SumI2OutMax=[]  SumI3OutMin=[]  SumI3OutMax=[]  SumI4OutMin=[]  SumI4OutMax=[]  SumDOutMin=[]  SumDOutMax=[]  DifferentiatorOutMin=[]  DifferentiatorOutMax=[]  FilterDiffOutCoefMin=[]  FilterDiffOutCoefMax=[]  ReciprocalOutMin=[]  ReciprocalOutMax=[]  SumDenOutMin=[]  SumDenOutMax=[]  SumNumOutMin=[]  SumNumOutMax=[]  DivideOutMin=[]  DivideOutMax=[]  UdiffTsProdOutMin=[]  UdiffTsProdOutMax=[]  NTsProdOutMin=[]  NTsProdOutMax=[]  UintegralTsProdOutMin=[]  UintegralTsProdOutMax=[]  UngainTsProdOutMin=[]  UngainTsProdOutMax=[]  ClampingZeroOutDataTypeStr=Inherit: Inherit via back propagation  ClampingZeroOutMin=[]  ClampingZeroOutMax=[]  FilterDenConstantOutDataTypeStr=Inherit: Inherit via back propagation  FilterDenConstantOutMin=[]  FilterDenConstantOutMax=[]  PCopyOutDataTypeStr=Inherit: Inherit via back propagation  PCopyOutMin=[]  PCopyOutMax=[]  NCopyOutDataTypeStr=Inherit: Inherit via back propagation  NCopyOutMin=[]  NCopyOutMax=[]  IntegratorContinuousStateAttributes=''  IntegratorStateMustResolveToSignalObject=off  IntegratorRTWStateStorageClass=Auto  FilterContinuousStateAttributes=''  FilterStateMustResolveToSignalObject=off  FilterRTWStateStorageClass=Auto  ParallelPVariant=InternalParameters  IdealPVariant=Disabled  IVariant=InternalParameters  DVariant=InternalParameters  IntegratorVariant=Continuous  SatVariant=Enabled  AWVariant=ContClampingParallel  PCopyVariant=Disabled  TRVariant=Disabled  FdbkBlocksVariant=Forward  IdealPFdbkVariant=Disabled  SatFdbkVariant=Disabled  DerivativeFilterVariant=ContFilter  NVariant=InternalParameters  NCopyVariant=Disabled  FilterICVariant=InternalICsFilter  IntegratorICVariant=InternalICs  ExternalResetVariant=Disabled  TRSumVariant=Passthrough  SumFdbkVariant=Disabled  SumVariant=Sum_PID  TsampFilterVariant=InternalTs  TsampNgainVariant=Passthrough  TsampIntegralVariant=Disabled_SignalSpec  ExternalSaturationOutDataTypeStr=Inherit: Same as second input  DerivativeSourceVariant=ErrorSignal  PreIntVariant=InternalPreInt
  Saturation1 : Saturate  UpperLimit=2  LowerLimit=-2
  Scope : Scope  NumInputPorts=2
  Scope1 : Scope  NumInputPorts=2
  Scope2 : Scope
  Sum1 : Sum  Inputs=|-+
  Sum4 : Sum  Inputs=|-+
  Terminator{,1..3} (4 alike) : Terminator
  dt : Outport
  wires:
  Demux6/3 -> Sum1/1, Gain5/1
  h_c/1 -> Scope1/2, Gain/1
  Ve/1 -> Demux5/1
  Demux5/2 -> Terminator1/1
  Demux6/1 -> Terminator2/1
  Demux5/1 -> Terminator/1
  Xe/1 -> Demux6/1
  Demux5/3 -> Sum4/1, Scope/1  "Vz"
  Sum1/1 -> PID Controller/1
  Demux6/2 -> Terminator3/1
  Gain/1 -> Sum1/2
  PID Controller/1 -> Saturation1/1  "Vzc"
  Gain5/1 -> Scope1/1  "h"
  PID Controller2/1 -> Gain4/1, Scope2/1
  Sum4/1 -> PID Controller2/1
  Gain4/1 -> dt/1
  Saturation1/1 -> Sum4/2, Scope/2  "Vz_c"
